simulink model "Integration_Forward_Forger_Line_Search"  (R2015a)
settings: Solver=ode3  StartTime=0.0  StopTime=T_opt  FixedStep=0.01  MaxStep=0.01  RelTol=1e-3
values from neighbouring files (symbols this model uses):
  I_update = I    [Gradient_Descent_Greedy_3rd.m]
  n0 = Periodic_Solution(time_shift(j)*100+1,4)    [Gradient_Descent_Greedy_3rd.m]
  Periodic_Solution = Periodic_Solution(101:end,:)    [Gradient_Descent_Greedy_3rd.m]    (also in Periodic_Solution_JFK_1000lux.mat = [0 0.00999999999999 0.02 0.03 0.04 0.05 0.0599999999999 0.06)
  T_opt = x(end,1)    [Gradient_Descent_Greedy_3rd.m]
  tol = 0.01    [Gradient_Descent_Greedy_3rd.m]
  x0 = Periodic_Solution(time_shift(j)*100+1,2)    [Gradient_Descent_Greedy_3rd.m]
  xc0 = Periodic_Solution(time_shift(j)*100+1,3)    [Gradient_Descent_Greedy_3rd.m]
settings Model: Creator=wangf7  LastModifiedBy=Jiawei Yin
settings OptimizationCC: ExpressionDepthLimit=2147483647
settings DebuggingCC: UnderspecifiedInitializationDetection=Classic  MergeDetectMultiDrivingBlocksExec=none  SolverPrmCheckMsg=warning  StateNameClashWarn=warning

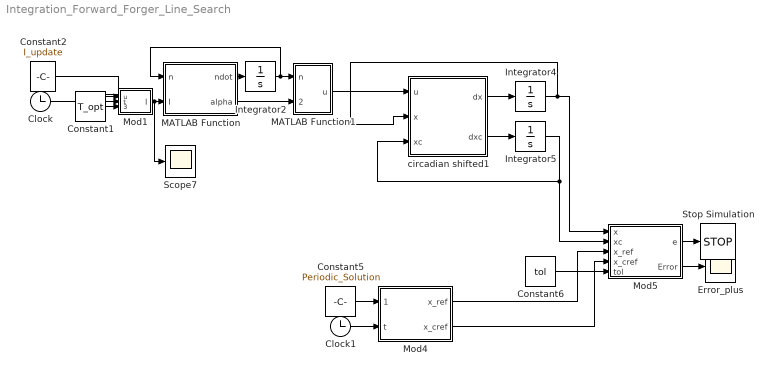
== system Integration_Forward_Forger_Line_Search ==
  Clock : Clock
  Clock1 : Clock
  Constant1 : Constant  Value=T_opt
  Constant2 : Constant  Value=I_update
  Constant5 : Constant  Value=Periodic_Solution
  Constant6 : Constant  Value=tol
  Error_plus : Scope
      settings: TimeRange=auto  MaxDataPoints=50000000  SaveName=Error_plus  YMin=-0.12715  YMax=0.13151  SampleTime=-1  DataFormat=Array
  Integrator2 : Integrator  InitialCondition=n0
  Integrator4 : Integrator  InitialCondition=x0
  Integrator5 : Integrator  InitialCondition=xc0
  MATLAB Function : MATLAB Function  TreatAsAtomicUnit=on
      settings: PermitHierarchicalResolution=ParametersOnly
  MATLAB Function1 : MATLAB Function  TreatAsAtomicUnit=on
      settings: PermitHierarchicalResolution=ParametersOnly
  Mod1 : MATLAB Function  TreatAsAtomicUnit=on
      settings: PermitHierarchicalResolution=ParametersOnly
  Mod4 : MATLAB Function  TreatAsAtomicUnit=on
      settings: PermitHierarchicalResolution=ParametersOnly
  Mod5 : MATLAB Function  TreatAsAtomicUnit=on
      settings: PermitHierarchicalResolution=ParametersOnly
  Scope7 : Scope
      settings: TimeRange=auto  MaxDataPoints=50000000  SaveName=I_plus  YMin=-0.12715  YMax=0.13151  SampleTime=-1  DataFormat=Array
  Stop Simulation : Stop
  circadian shifted1 : MATLAB Function  TreatAsAtomicUnit=on
      settings: PermitHierarchicalResolution=ParametersOnly
  wires:
  circadian shifted1/1(dx) -> Integrator4/1
  circadian shifted1/2(dxc) -> Integrator5/1
  Integrator4/1 -> circadian shifted1/2(x), Mod5/1(x)
  Clock/1 -> Mod1/2(t)
  Constant2/1 -> Mod1/1(u)
  Integrator5/1 -> Mod5/2(xc), circadian shifted1/3(xc)
  Constant5/1 -> Mod4/1(Periodic_Solution)
  Clock1/1 -> Mod4/2(t)
  Mod5/1(e) -> Stop Simulation/1
  Mod4/1(x_ref) -> Mod5/3(x_ref)
  Mod4/2(x_cref) -> Mod5/4(x_cref)
  Constant6/1 -> Mod5/5(tol)
  Constant1/1 -> Mod1/3(T_opt)
  MATLAB Function/1(ndot) -> Integrator2/1
  Integrator2/1 -> MATLAB Function/1(n), MATLAB Function1/1(n)
  MATLAB Function/2(alpha) -> MATLAB Function1/2(alpha)
  Mod1/1(I) -> Scope7/1, MATLAB Function/2(I)
  MATLAB Function1/1(u) -> circadian shifted1/1(u)
  Mod5/2(Error) -> Error_plus/1

== matlab function Integration_Forward_Forger_Line_Search/MATLAB Function ==
  data: n input; I input; ndot output; alpha output
function [ndot,alpha] = fcn(n,I)

alpha0=0.05;
beta=0.0075;
I0=9500;
alpha=alpha0*(I/I0)^0.5;
ndot=60*[alpha*(1-n)-beta*n];

== matlab function Integration_Forward_Forger_Line_Search/Mod1 ==
  data: u input; I output; t input; T_opt input
function I  = fcn(u,t,T_opt)
%#codegen
if t<=T_opt
    I=interp1q(u(:,1),u(:,2),t);
else
    I=u(end,2);
end

== matlab function Integration_Forward_Forger_Line_Search/circadian shifted1 ==
  data: u input; x input; xc input; dx output; dxc output
function [dx,dxc] = fcn(u,x,xc)

k=0.55;
mu=0.13;
q=1/3;
B=(1-0.4*x)*(1-0.4*xc)*u;
tau=24.2;

dx = pi*(xc+mu*(x/3+4*x^3/3-256*x^7/105)+B)/12;
dxc = pi*(q*B*xc-x*((24/0.99729/tau)^2+k*B))/12;

== matlab function Integration_Forward_Forger_Line_Search/Mod4 ==
  data: Periodic_Solution input; x_ref output; t input; x_cref output
function [x_ref,x_cref] = fcn(Periodic_Solution,t)
%#codegen
x_ref=interp1q(Periodic_Solution(:,1),Periodic_Solution(:,2),t);
x_cref=interp1q(Periodic_Solution(:,1),Periodic_Solution(:,3),t);

== matlab function Integration_Forward_Forger_Line_Search/Mod5 ==
  data: x input; xc input; e output; x_ref input; x_cref input; tol input; Error output
function [e,Error] = fcn(x,xc,x_ref,x_cref,tol)
%#codege
Error=(x-x_ref)^2+(xc-x_cref)^2;
e=Error<tol;

== matlab function Integration_Forward_Forger_Line_Search/MATLAB Function1 ==
  data: n input; u output; alpha input
function u = fcn(n,alpha)
%#codegen
u=33.75*alpha*(1-n);
